simulink model "Robot"  (R2018a)
settings: Solver=VariableStepAuto  StartTime=0.0  StopTime=inf  FixedStep=1e-4  RelTol=1e-3  EnableMultiTasking=on
values from neighbouring files (symbols this model uses):
  CM730_acc_center = (4 * 9.80665)    (= 39.2266)    [CM730.m]
  CM730_acc_gain = 512 / CM730_acc_center    (= 13.0523675261)    [CM730.m]
  CM730_gyro_center = (1600 / 360 * 2 * pi)    (= 27.9252680319)    [CM730.m]
  CM730_gyro_gain = 512 / CM730_gyro_center    (= 18.3346494442)    [CM730.m]
  CM730_sample_time = 1e-3    (= 0.001)    [CM730.m]
  FSR_max = 254    [FSR.m]
  FSR_no_load = 255    [FSR.m]
  FSR_sample_time = 0.001    [FSR.m]
  FSR_scale = 1000    [FSR.m]
  g = 0    [Euler.m]
  MX106_Te = 1/1000    (= 0.001)    [MX106_init.m]
  MX28_inertia = 9e-8 * MX28_reduction^2    (= 0.0033385284)    [MX28_init.m]
  MX28_Te = 1/1000    (= 0.001)    [MX28_init.m]
  posZero_ID1 = posZero(1)    [Robot_init.m]
  posZero_ID10 = posZero(14)    [Robot_init.m]
  posZero_ID11 = posZero(9)    [Robot_init.m]
  posZero_ID12 = posZero(15)    [Robot_init.m]
  posZero_ID13 = posZero(10)    [Robot_init.m]
  posZero_ID14 = posZero(16)    [Robot_init.m]
  posZero_ID15 = posZero(11)    [Robot_init.m]
  posZero_ID16 = posZero(17)    [Robot_init.m]
  posZero_ID17 = posZero(12)    [Robot_init.m]
  posZero_ID18 = posZero(18)    [Robot_init.m]
  posZero_ID19 = posZero(19)    [Robot_init.m]
  posZero_ID2 = posZero(4)    [Robot_init.m]
  posZero_ID20 = posZero(20)    [Robot_init.m]
  posZero_ID3 = posZero(2)    [Robot_init.m]
  posZero_ID4 = posZero(5)    [Robot_init.m]
  posZero_ID5 = posZero(3)    [Robot_init.m]
  posZero_ID6 = posZero(6)    [Robot_init.m]
  posZero_ID7 = posZero(7)    [Robot_init.m]
  posZero_ID8 = posZero(13)    [Robot_init.m]
  posZero_ID9 = posZero(8)    [Robot_init.m]
  robot_chest_mass = 2385.0    (= 2385)    [Robot_init.m]
  robot_floor_friction_coeff = 0.6    [Robot_init.m]
  robot_floor_position_gain = -1e5    (= -100000)    [Robot_init.m]
  robot_floor_speed_gain = -1e3    (= -1000)    [Robot_init.m]
  robot_gravity = [0 0 0]    [Robot_init.m]
  robot_head_mass = 177.69    [Robot_init.m]
  robot_hip1_mass = 49.00    (= 49)    [Robot_init.m]
  robot_left_ankle_mass = 360.00    (= 360)    [Robot_init.m]
  robot_left_foot_mass = 267.00    (= 267)    [Robot_init.m]
  robot_left_forearm_mass = 248.00    (= 248)    [Robot_init.m]
  robot_left_hip2_mass = 358.00    (= 358)    [Robot_init.m]
  robot_left_lower_leg_mass = 129.00    (= 129)    [Robot_init.m]
  robot_left_shoulder_mass = 39.00    (= 39)    [Robot_init.m]
  robot_left_thigh_mass = 1263.00    (= 1263)    [Robot_init.m]
  robot_left_upper_arm_mass = 247.00    (= 247)    [Robot_init.m]
  robot_neck_mass = 90    [Robot_init.m]
  robot_right_ankle_mass = 360.00    (= 360)    [Robot_init.m]
  robot_right_foot_mass = 267.00    (= 267)    [Robot_init.m]
  robot_right_forearm_mass = 248.00    (= 248)    [Robot_init.m]
  robot_right_hip2_mass = 358.00    (= 358)    [Robot_init.m]
  robot_right_lower_leg_mass = 129.00    (= 129)    [Robot_init.m]
  robot_right_shoulder_mass = 39.00    (= 39)    [Robot_init.m]
  robot_right_thigh_mass = 263.00    (= 263)    [Robot_init.m]
  robot_right_upper_arm_mass = 247.00    (= 247)    [Robot_init.m]
  X = get(hObject,'Value')    [gui_kine.m]
  Y = get(hObject,'Value')    [gui_kine.m]
  Z = get(hObject,'Value')    [gui_kine.m]
libraries: sm_lib x167, fl_lib x128, nesl_utility x77, dspindex x1
(part 6 of 7)

== system Robot/Robot simulation/Right Leg/Right Knee (13) ==
  Inertia : sm_lib/Body Elements/Inertia  InertiaType=Custom  Mass=1  MassUnits=g  CenterOfMass=[0 0 0]  CenterOfMassUnits=m  MomentsOfInertia=[0 0 MX28_inertia]  MomentsOfInertiaUnits=kg*m^2  ProductsOfInertia=[0 0 0]  ProductsOfInertiaUnits=kg*m^2  GraphicType=Marker  MarkerShape=Inertia  MarkerSize=20  GraphicVisPropType=SimpleVisualProperties  GraphicDiffuseColor=[0.5 0.5 0.5]  GraphicSpecularColor=[0.5 0.5 0.5 1.0]  GraphicAmbientColor=[0.15 0.15 0.15 1.0]  GraphicEmissiveColor=[0.0 0.0 0.0 1.0]  GraphicShininess=75  GraphicOpacity=1.0
  MX106 Command : DataStoreRead  DataStoreName=MX106_ID13  SampleTime=MX106_Te  DataStoreElements=MX106_ID13.CW_angle_limit#MX106_ID13.CCW_angle_limit#MX106_ID13.torque_enable#MX106_ID13.D_gain#MX106_ID13.I_gain#MX106_ID13.P_gain#MX106_ID13.goal_position#MX106_ID13.moving_speed#MX106_ID13.torque_limit
  MX106 State : DataStoreWrite  DataStoreName=MX106_ID13  DataStoreElements=MX106_ID13.present_position#MX106_ID13.present_speed#MX106_ID13.present_load#MX106_ID13.moving#MX106_ID13.pwm
  Model : ModelReference  ModelNameDialog=MX106.slx  SimulationMode=Normal  ModelReferenceVersion=1.67
  Position converter : nesl_utility/PS-Simulink Converter  PhysicalDomain=network_engine_domain  SubClassName=ps_output  LeftPortType=input  RightPortType=output  PseudoPeriodic=off  Frequencies=[]  Unit=rad  AffineConversion=off
  Revolute Joint : sm_lib/Joints/Revolute Joint  SenseConstraintForce=off  SenseConstraintForceX=off  SenseConstraintForceY=off  SenseConstraintForceZ=off  SenseConstraintTorque=off  SenseConstraintTorqueX=off  SenseConstraintTorqueY=off  SenseConstraintTorqueZ=off  SenseTotalForce=off  SenseTotalForceX=off  SenseTotalForceY=off  SenseTotalForceZ=off  SenseTotalTorque=off  SenseTotalTorqueX=off  SenseTotalTorqueY=off  SenseTotalTorqueZ=off  CompositeWrenchDir=FollowerOnBase  CompositeWrenchFrame=BaseFrame  EquilibriumPosition=0  EquilibriumPositionUnits=deg  SpringStiffness=0  SpringStiffnessUnits=N*m/deg  DampingCoefficient=MX28_lub_friction  DampingCoefficientUnits=N*m/(rad/s)  TorqueActuationMode=InputTorque  MotionActuationMode=ComputedMotion  SensePosition=on  SenseVelocity=on  SenseAcceleration=off  SenseTorqueForce=off  PositionTargetSpecify=on  PositionTargetPriority=High  PositionTargetValue=MX28_init_position  PositionTargetValueUnits=rad  VelocityTargetSpecify=on  VelocityTargetPriority=High  VelocityTargetValue=MX28_init_speed  VelocityTargetValueUnits=rad/s
  Speed converter : nesl_utility/PS-Simulink Converter  PhysicalDomain=network_engine_domain  SubClassName=ps_output  LeftPortType=input  RightPortType=output  PseudoPeriodic=off  Frequencies=[]  Unit=rad/s  AffineConversion=off
  Torque converter : nesl_utility/Simulink-PS Converter  PhysicalDomain=network_engine_domain  SubClassName=ps_input  LeftPortType=input  RightPortType=output  PseudoPeriodic=off  Frequencies=[]  NoiseDistribution=none  NoiseParameters=[]  Unit=N*m  AffineConversion=off  FilteringAndDerivatives=zero  SimscapeFilterOrder=1  InputFilterTimeConstant=0.001  UdotUserProvided=1
  Base : PMIOPort  Side=Left
  Axis : PMIOPort  Port=2  Side=Right
  wires:
  Model/4 -> MX106 State/3
  Model/2 -> MX106 State/1
  Model/5 -> MX106 State/4
  Model/3 -> MX106 State/2
  MX106 Command/3 -> Model/5
  MX106 Command/6 -> Model/8
  MX106 Command/4 -> Model/6
  MX106 Command/5 -> Model/7
  MX106 Command/7 -> Model/9
  MX106 Command/2 -> Model/4
  MX106 Command/1 -> Model/3
  Position converter/1 -> Model/2
  Speed converter/1 -> Model/1
  Model/6 -> MX106 State/5
  MX106 Command/8 -> Model/10
  MX106 Command/9 -> Model/11
  Model/1 -> Torque converter/1
  connections:
  Axis/RConn1 -- Revolute Joint/RConn1 -- Inertia/RConn1
  Revolute Joint/LConn1 -- Base/RConn1
  Revolute Joint/RConn3 -- Speed converter/LConn1
  Revolute Joint/RConn2 -- Position converter/LConn1
  Revolute Joint/LConn2 -- Torque converter/RConn1

== system Robot/Robot simulation/Right Leg/Right Lower Leg ==
  Right Lower Leg Axis to Right Ankle Axis : sm_lib/Frames and Transforms/Rigid Transform  TranslationMethod=Cartesian  TranslationStandardOffset=0  TranslationLengthUnit=mm  TranslationStandardAxis=+Z  TranslationCartesianOffset=robot_right_lower_leg_to_right_ankle_tra  TranslationROffset=0  TranslationROffsetUnits=m  TranslationZOffset=0  TranslationZOffsetUnits=m  TranslationThetaOffset=0  TranslationThetaOffsetUnits=deg  RotationMethod=RotationMatrix  RotationAngleUnits=deg  RotationStandardAxis=+Z  RotationAngle=0  RotationArbitraryAxis=[0 0 1]  FollAlignAxisA=+X  BaseAlignAxisA=+Y  FollAlignAxisB=+Y  BaseAlignAxisB=+Z  RotationSequenceAxes=FollowerAxes  RotationSequence=XYX  RotationSequenceAngles=[0 0 0]  RotationSequenceAnglesUnits=deg  RotationMatrix=robot_right_lower_leg_to_right_ankle_rot
  Solid : sm_lib/Body Elements/Solid  InertiaType=Custom  Mass=robot_right_lower_leg_mass  MassUnits=g  CenterOfMass=robot_right_lower_leg_to_center_mass  CenterOfMassUnits=mm  MomentsOfInertia=robot_right_lower_leg_moment_inertia  MomentsOfInertiaUnits=g*mm^2  ProductsOfInertia=robot_right_lower_leg_product_inertia  ProductsOfInertiaUnits=g*mm^2  DensityBased=on  Density=1000  DensityUnits=kg/(m^3)  DoExposeReferenceFrame=on  SerializedFrames=<Frames/>  GraphicType=FromGeometry  MarkerShape=Sphere  MarkerSize=10  MarkerSizeUnits=m  GraphicVisPropType=SimpleVisualProperties  GraphicDiffuseColor=[0.5 0.5 0.5]  GraphicSpecularColor=[0.5 0.5 0.5 1.0]  GraphicAmbientColor=[0.15 0.15 0.15 1.0]  GraphicEmissiveColor=[0.0 0.0 0.0 1.0]  GraphicShininess=75  GraphicOpacity=1.0  GeometryShape=FromFile  RectangleSize=[1 1]  RectangleSizeUnits=m  BrickDimensions=[1 1 1]  BrickDimensionUnits=m  CylinderRadius=1  CylinderRadiusUnits=m  CylinderLength=1  CylinderLengthUnits=m  SphereRadius=1  SphereRadiusUnits=m  EllipsoidRadii=[1 1 1]  EllipsoidRadiiUnits=m  ExtrusionCrossSection=[1 1; -1 1; -1 -1; 1 -1]  ExtrusionCrossSectionUnits=m  ExtrusionLength=1  ExtrusionLengthUnits=m  PolygonNumSides=3  PolygonOuterRadius=1  PolygonOuterRadiusUnits=m  ExtGeomFileType=STL  ExtGeomFileName=\STL\Right_Lower_Leg.STL  ExtGeomFileUnits=mm  RevolutionCrossSection=[1 1; 1 -1; 2 -1; 2 1]  RevolutionCrossSectionUnits=m  RevolutionExtent=Full  RevolutionAngle=180  RevolutionAngleUnits=deg
  Right Knee : PMIOPort  Side=Left
  Right Ankle Pitch : PMIOPort  Port=2  Side=Right
  connections:
  Solid/RConn1 -- Right Lower Leg Axis to Right Ankle Axis/LConn1 -- Right Knee/RConn1
  Right Ankle Pitch/RConn1 -- Right Lower Leg Axis to Right Ankle Axis/RConn1

== system Robot/Robot simulation/Right Leg/Right Thigh ==
  Right Hip Pitch Axis to Right Lower Leg Base : sm_lib/Frames and Transforms/Rigid Transform  TranslationMethod=Cartesian  TranslationStandardOffset=0  TranslationLengthUnit=mm  TranslationStandardAxis=+Z  TranslationCartesianOffset=robot_right_thigh_to_right_lower_leg_tra  TranslationROffset=0  TranslationROffsetUnits=m  TranslationZOffset=0  TranslationZOffsetUnits=m  TranslationThetaOffset=0  TranslationThetaOffsetUnits=deg  RotationMethod=RotationMatrix  RotationAngleUnits=deg  RotationStandardAxis=+Z  RotationAngle=0  RotationArbitraryAxis=[0 0 1]  FollAlignAxisA=+X  BaseAlignAxisA=+Y  FollAlignAxisB=+Y  BaseAlignAxisB=+Z  RotationSequenceAxes=FollowerAxes  RotationSequence=XYX  RotationSequenceAngles=[0 0 0]  RotationSequenceAnglesUnits=deg  RotationMatrix=robot_right_thigh_to_right_lower_leg_rot
  Solid : sm_lib/Body Elements/Solid  InertiaType=Custom  Mass=robot_right_thigh_mass  MassUnits=g  CenterOfMass=robot_right_thigh_to_center_mass  CenterOfMassUnits=mm  MomentsOfInertia=robot_right_thigh_moment_inertia  MomentsOfInertiaUnits=g*mm^2  ProductsOfInertia=robot_right_thigh_product_inertia  ProductsOfInertiaUnits=g*mm^2  DensityBased=on  Density=1000  DensityUnits=kg/(m^3)  DoExposeReferenceFrame=on  SerializedFrames=<Frames/>  GraphicType=FromGeometry  MarkerShape=Sphere  MarkerSize=10  MarkerSizeUnits=m  GraphicVisPropType=SimpleVisualProperties  GraphicDiffuseColor=[0.5 0.5 0.5]  GraphicSpecularColor=[0.5 0.5 0.5 1.0]  GraphicAmbientColor=[0.15 0.15 0.15 1.0]  GraphicEmissiveColor=[0.0 0.0 0.0 1.0]  GraphicShininess=75  GraphicOpacity=1.0  GeometryShape=FromFile  RectangleSize=[1 1]  RectangleSizeUnits=m  BrickDimensions=[1 1 1]  BrickDimensionUnits=m  CylinderRadius=1  CylinderRadiusUnits=m  CylinderLength=1  CylinderLengthUnits=m  SphereRadius=1  SphereRadiusUnits=m  EllipsoidRadii=[1 1 1]  EllipsoidRadiiUnits=m  ExtrusionCrossSection=[1 1; -1 1; -1 -1; 1 -1]  ExtrusionCrossSectionUnits=m  ExtrusionLength=1  ExtrusionLengthUnits=m  PolygonNumSides=3  PolygonOuterRadius=1  PolygonOuterRadiusUnits=m  ExtGeomFileType=STL  ExtGeomFileName=\STL\Right_Thigh.STL  ExtGeomFileUnits=mm  RevolutionCrossSection=[1 1; 1 -1; 2 -1; 2 1]  RevolutionCrossSectionUnits=m  RevolutionExtent=Full  RevolutionAngle=180  RevolutionAngleUnits=deg
  Right Hip Pitch : PMIOPort  Side=Left
  Right Knee : PMIOPort  Port=2  Side=Right
  connections:
  Right Hip Pitch Axis to Right Lower Leg Base/LConn1 -- Right Hip Pitch/RConn1 -- Solid/RConn1
  Right Knee/RConn1 -- Right Hip Pitch Axis to Right Lower Leg Base/RConn1

== system Robot/Robot simulation/Left Leg/Floor model/Floor Model Back Left ==
  6-DOF Joint1 : sm_lib/Joints/6-DOF Joint  SenseConstraintForce=off  SenseConstraintForceX=off  SenseConstraintForceY=off  SenseConstraintForceZ=off  SenseConstraintTorque=off  SenseConstraintTorqueX=off  SenseConstraintTorqueY=off  SenseConstraintTorqueZ=off  SenseTotalForce=off  SenseTotalForceX=off  SenseTotalForceY=off  SenseTotalForceZ=off  SenseTotalTorque=off  SenseTotalTorqueX=off  SenseTotalTorqueY=off  SenseTotalTorqueZ=off  CompositeWrenchDir=FollowerOnBase  CompositeWrenchFrame=BaseFrame  PxEquilibriumPosition=0  PxEquilibriumPositionUnits=m  PxSpringStiffness=0  PxSpringStiffnessUnits=N/m  PxDampingCoefficient=0  PxDampingCoefficientUnits=N/(m/s)  PxTorqueActuationMode=InputTorque  PxMotionActuationMode=ComputedMotion  PxSensePosition=off  PxSenseVelocity=on  PxSenseAcceleration=off  PxSenseTorqueForce=off  PxPositionTargetSpecify=off  PxPositionTargetPriority=High  PxPositionTargetValue=0  PxPositionTargetValueUnits=m  PxVelocityTargetSpecify=off  PxVelocityTargetPriority=High  PxVelocityTargetValue=0  PxVelocityTargetValueUnits=m/s  PyEquilibriumPosition=0  PyEquilibriumPositionUnits=m  PySpringStiffness=0  PySpringStiffnessUnits=N/m  PyDampingCoefficient=0  PyDampingCoefficientUnits=N/(m/s)  PyTorqueActuationMode=InputTorque  PyMotionActuationMode=ComputedMotion  PySensePosition=off  PySenseVelocity=on  PySenseAcceleration=off  PySenseTorqueForce=off  PyPositionTargetSpecify=off  PyPositionTargetPriority=High  PyPositionTargetValue=0  PyPositionTargetValueUnits=m  PyVelocityTargetSpecify=off  PyVelocityTargetPriority=High  PyVelocityTargetValue=0  PyVelocityTargetValueUnits=m/s  PzEquilibriumPosition=0  PzEquilibriumPositionUnits=m  PzSpringStiffness=0  PzSpringStiffnessUnits=N/m  PzDampingCoefficient=0  PzDampingCoefficientUnits=N/(m/s)  PzTorqueActuationMode=InputTorque  PzMotionActuationMode=ComputedMotion  PzSensePosition=on  PzSenseVelocity=on  PzSenseAcceleration=off  PzSenseTorqueForce=off  PzPositionTargetSpecify=off  PzPositionTargetPriority=High  PzPositionTargetValue=0  PzPositionTargetValueUnits=m  PzVelocityTargetSpecify=off  PzVelocityTargetPriority=High  PzVelocityTargetValue=0  PzVelocityTargetValueUnits=m/s  SphDefPosRotationMethod=None  SphDefPosRotationAngleUnits=deg  SphDefPosRotationStandardAxis=+Z  SphDefPosRotationAngle=0.0  SphDefPosRotationArbitraryAxis=[0 0 1]  SphDefPosFollAlignAxisA=+X  SphDefPosBaseAlignAxisA=+Y  SphDefPosFollAlignAxisB=+Y  SphDefPosBaseAlignAxisB=+Z  SphDefPosRotationSequenceAxes=FollowerAxes  SphDefPosRotationSequence=XYX  SphDefPosRotationSequenceAngles=[0 0 0]  SphDefPosRotationSequenceAnglesUnits=deg  SphDefPosRotationMatrix=[1 0 0; 0 1 0; 0 0 1]  SphEqPosRotationMethod=None  SphEqPosRotationAngleUnits=deg  SphEqPosRotationStandardAxis=+Z  SphEqPosRotationAngle=0.0  SphEqPosRotationArbitraryAxis=[0 0 1]  SphEqPosFollAlignAxisA=+X  SphEqPosBaseAlignAxisA=+Y  SphEqPosFollAlignAxisB=+Y  SphEqPosBaseAlignAxisB=+Z  SphEqPosRotationSequenceAxes=FollowerAxes  SphEqPosRotationSequence=XYX  SphEqPosRotationSequenceAngles=[0 0 0]  SphEqPosRotationSequenceAnglesUnits=deg  SphEqPosRotationMatrix=[1 0 0; 0 1 0; 0 0 1]  SphSpringStiffness=0  SphSpringStiffnessUnits=N*m/deg  SphDampingCoefficient=0  SphDampingCoefficientUnits=N*m/(deg/s)  SphActuateTorqueX=off  SphActuateTorqueY=off  SphActuateTorqueZ=off  SphActuateTorque=off  SphTorqueActuationMode=NoTorque  SphMotionActuationMode=ComputedMotion  SphActuationFrame=BaseFrame  SphSensePosition=off  SphSenseVelocityX=off  SphSenseVelocityY=off  SphSenseVelocityZ=off  SphSenseVelocity=off  SphSenseAccelerationX=off  SphSenseAccelerationY=off  SphSenseAccelerationZ=off  SphSenseAcceleration=off  SphSenseTorqueX=off  SphSenseTorqueY=off  SphSenseTorqueZ=off  SphSenseTorqueForce=off  SphSensingFrame=BaseFrame  SphPositionTargetRotationMethod=None  SphPositionTargetRotationAngleUnits=deg  SphPositionTargetRotationStandardAxis=+Z  SphPositionTargetRotationAngle=0.0  SphPositionTargetRotationArbitraryAxis=[0 0 1]  SphPositionTargetFollAlignAxisA=+X  SphPositionTargetBaseAlignAxisA=+Y  SphPositionTargetFollAlignAxisB=+Y  SphPositionTargetBaseAlignAxisB=+Z  SphPositionTargetRotationSequenceAxes=FollowerAxes  SphPositionTargetRotationSequence=XYX  SphPositionTargetRotationSequenceAngles=[0 0 0]  SphPositionTargetRotationSequenceAnglesUnits=deg  SphPositionTargetRotationMatrix=[1 0 0; 0 1 0; 0 0 1]  SphPositionTargetSpecify=off  SphPositionTargetPriority=High  SphVelocityTargetValue=[0 0 0]  SphVelocityTargetValueUnits=deg/s  SphVelocityTargetSpecify=off  SphVelocityTargetPriority=High  SphVelocityTargetInFollowerFrame=on
  Friction coeff : fl_lib/Physical Signals/Functions/PS Gain  gain=robot_floor_friction_coeff
  No friction : fl_lib/Physical Signals/Sources/PS Constant  constant=0
  PS Abs : fl_lib/Physical Signals/Nonlinear Operators/PS Abs
      settings: SourceProductName=Simscape  SourceProductBaseCode=SS
  PS-Simulink Converter : nesl_utility/PS-Simulink Converter  PhysicalDomain=network_engine_domain  SubClassName=ps_output  LeftPortType=input  RightPortType=output  PseudoPeriodic=off  Frequencies=[]  Unit=N  AffineConversion=off
  Saturation : Saturate  UpperLimit=+inf  LowerLimit=0
  Unary minus : fl_lib/Physical Signals/Functions/PS Gain  gain=-1
  X Lower Bound : fl_lib/Physical Signals/Nonlinear Operators/PS Max
      settings: SourceProductName=Simscape  SourceProductBaseCode=SS
  X Speed Gain : fl_lib/Physical Signals/Functions/PS Gain  gain=robot_floor_speed_gain
  X Switch : fl_lib/Physical Signals/Nonlinear Operators/PS Switch  Threshold=0
      settings: SourceProductName=Simscape  SourceProductBaseCode=SS
  X Upper Bound : fl_lib/Physical Signals/Nonlinear Operators/PS Min
      settings: SourceProductName=Simscape  SourceProductBaseCode=SS
  Y Lower Bound : fl_lib/Physical Signals/Nonlinear Operators/PS Max
      settings: SourceProductName=Simscape  SourceProductBaseCode=SS
  Y Speed Gain : fl_lib/Physical Signals/Functions/PS Gain  gain=robot_floor_speed_gain
  Y Switch : fl_lib/Physical Signals/Nonlinear Operators/PS Switch  Threshold=0
      settings: SourceProductName=Simscape  SourceProductBaseCode=SS
  Y Upper Bound : fl_lib/Physical Signals/Nonlinear Operators/PS Min
      settings: SourceProductName=Simscape  SourceProductBaseCode=SS
  Z Add : fl_lib/Physical Signals/Functions/PS Add
  Z Position Gain : fl_lib/Physical Signals/Functions/PS Gain  gain=robot_floor_position_gain
  Z Speed Gain : fl_lib/Physical Signals/Functions/PS Gain  gain=robot_floor_speed_gain
  Z Switch : fl_lib/Physical Signals/Nonlinear Operators/PS Switch  Threshold=0
      settings: SourceProductName=Simscape  SourceProductBaseCode=SS
  Contact : PMIOPort  Side=Left
  Floor : PMIOPort  Port=2  Side=Right
  Z force : Outport
  wires:
  PS-Simulink Converter/1 -> Saturation/1
  Saturation/1 -> Z force/1
  connections:
  Floor/RConn1 -- 6-DOF Joint1/LConn1
  6-DOF Joint1/RConn1 -- Contact/RConn1
  No friction/RConn1 -- Y Switch/LConn1 -- Z Switch/LConn1 -- X Switch/LConn1
  Z Position Gain/RConn1 -- Z Add/LConn1
  Z Switch/LConn3 -- Z Add/RConn1 -- Friction coeff/LConn1 -- PS-Simulink Converter/LConn1
  Z Speed Gain/RConn1 -- Z Add/LConn2
  6-DOF Joint1/RConn5 -- Z Speed Gain/LConn1
  6-DOF Joint1/LConn4 -- Z Switch/RConn1
  Z Switch/LConn2 -- Z Position Gain/LConn1 -- 6-DOF Joint1/RConn4 -- X Switch/LConn2 -- Y Switch/LConn2
  Y Switch/RConn1 -- 6-DOF Joint1/LConn3
  Y Speed Gain/LConn1 -- 6-DOF Joint1/RConn3
  PS Abs/LConn1 -- Friction coeff/RConn1
  PS Abs/RConn1 -- Unary minus/LConn1 -- X Upper Bound/LConn2 -- Y Upper Bound/LConn2
  Y Upper Bound/RConn1 -- Y Lower Bound/LConn1
  Y Lower Bound/LConn2 -- Unary minus/RConn1 -- X Lower Bound/LConn2
  Y Lower Bound/RConn1 -- Y Switch/LConn3
  Y Upper Bound/LConn1 -- Y Speed Gain/RConn1
  X Speed Gain/LConn1 -- 6-DOF Joint1/RConn2
  X Upper Bound/LConn1 -- X Speed Gain/RConn1
  X Lower Bound/LConn1 -- X Upper Bound/RConn1
  X Switch/LConn3 -- X Lower Bound/RConn1
  X Switch/RConn1 -- 6-DOF Joint1/LConn2

== system Robot/Robot simulation/Left Leg/Floor model/Floor Model Back Right ==
  6-DOF Joint1 : sm_lib/Joints/6-DOF Joint  SenseConstraintForce=off  SenseConstraintForceX=off  SenseConstraintForceY=off  SenseConstraintForceZ=off  SenseConstraintTorque=off  SenseConstraintTorqueX=off  SenseConstraintTorqueY=off  SenseConstraintTorqueZ=off  SenseTotalForce=off  SenseTotalForceX=off  SenseTotalForceY=off  SenseTotalForceZ=off  SenseTotalTorque=off  SenseTotalTorqueX=off  SenseTotalTorqueY=off  SenseTotalTorqueZ=off  CompositeWrenchDir=FollowerOnBase  CompositeWrenchFrame=BaseFrame  PxEquilibriumPosition=0  PxEquilibriumPositionUnits=m  PxSpringStiffness=0  PxSpringStiffnessUnits=N/m  PxDampingCoefficient=0  PxDampingCoefficientUnits=N/(m/s)  PxTorqueActuationMode=InputTorque  PxMotionActuationMode=ComputedMotion  PxSensePosition=off  PxSenseVelocity=on  PxSenseAcceleration=off  PxSenseTorqueForce=off  PxPositionTargetSpecify=off  PxPositionTargetPriority=High  PxPositionTargetValue=0  PxPositionTargetValueUnits=m  PxVelocityTargetSpecify=off  PxVelocityTargetPriority=High  PxVelocityTargetValue=0  PxVelocityTargetValueUnits=m/s  PyEquilibriumPosition=0  PyEquilibriumPositionUnits=m  PySpringStiffness=0  PySpringStiffnessUnits=N/m  PyDampingCoefficient=0  PyDampingCoefficientUnits=N/(m/s)  PyTorqueActuationMode=InputTorque  PyMotionActuationMode=ComputedMotion  PySensePosition=off  PySenseVelocity=on  PySenseAcceleration=off  PySenseTorqueForce=off  PyPositionTargetSpecify=off  PyPositionTargetPriority=High  PyPositionTargetValue=0  PyPositionTargetValueUnits=m  PyVelocityTargetSpecify=off  PyVelocityTargetPriority=High  PyVelocityTargetValue=0  PyVelocityTargetValueUnits=m/s  PzEquilibriumPosition=0  PzEquilibriumPositionUnits=m  PzSpringStiffness=0  PzSpringStiffnessUnits=N/m  PzDampingCoefficient=0  PzDampingCoefficientUnits=N/(m/s)  PzTorqueActuationMode=InputTorque  PzMotionActuationMode=ComputedMotion  PzSensePosition=on  PzSenseVelocity=on  PzSenseAcceleration=off  PzSenseTorqueForce=off  PzPositionTargetSpecify=off  PzPositionTargetPriority=High  PzPositionTargetValue=0  PzPositionTargetValueUnits=m  PzVelocityTargetSpecify=off  PzVelocityTargetPriority=High  PzVelocityTargetValue=0  PzVelocityTargetValueUnits=m/s  SphDefPosRotationMethod=None  SphDefPosRotationAngleUnits=deg  SphDefPosRotationStandardAxis=+Z  SphDefPosRotationAngle=0.0  SphDefPosRotationArbitraryAxis=[0 0 1]  SphDefPosFollAlignAxisA=+X  SphDefPosBaseAlignAxisA=+Y  SphDefPosFollAlignAxisB=+Y  SphDefPosBaseAlignAxisB=+Z  SphDefPosRotationSequenceAxes=FollowerAxes  SphDefPosRotationSequence=XYX  SphDefPosRotationSequenceAngles=[0 0 0]  SphDefPosRotationSequenceAnglesUnits=deg  SphDefPosRotationMatrix=[1 0 0; 0 1 0; 0 0 1]  SphEqPosRotationMethod=None  SphEqPosRotationAngleUnits=deg  SphEqPosRotationStandardAxis=+Z  SphEqPosRotationAngle=0.0  SphEqPosRotationArbitraryAxis=[0 0 1]  SphEqPosFollAlignAxisA=+X  SphEqPosBaseAlignAxisA=+Y  SphEqPosFollAlignAxisB=+Y  SphEqPosBaseAlignAxisB=+Z  SphEqPosRotationSequenceAxes=FollowerAxes  SphEqPosRotationSequence=XYX  SphEqPosRotationSequenceAngles=[0 0 0]  SphEqPosRotationSequenceAnglesUnits=deg  SphEqPosRotationMatrix=[1 0 0; 0 1 0; 0 0 1]  SphSpringStiffness=0  SphSpringStiffnessUnits=N*m/deg  SphDampingCoefficient=0  SphDampingCoefficientUnits=N*m/(deg/s)  SphActuateTorqueX=off  SphActuateTorqueY=off  SphActuateTorqueZ=off  SphActuateTorque=off  SphTorqueActuationMode=NoTorque  SphMotionActuationMode=ComputedMotion  SphActuationFrame=BaseFrame  SphSensePosition=off  SphSenseVelocityX=off  SphSenseVelocityY=off  SphSenseVelocityZ=off  SphSenseVelocity=off  SphSenseAccelerationX=off  SphSenseAccelerationY=off  SphSenseAccelerationZ=off  SphSenseAcceleration=off  SphSenseTorqueX=off  SphSenseTorqueY=off  SphSenseTorqueZ=off  SphSenseTorqueForce=off  SphSensingFrame=BaseFrame  SphPositionTargetRotationMethod=None  SphPositionTargetRotationAngleUnits=deg  SphPositionTargetRotationStandardAxis=+Z  SphPositionTargetRotationAngle=0.0  SphPositionTargetRotationArbitraryAxis=[0 0 1]  SphPositionTargetFollAlignAxisA=+X  SphPositionTargetBaseAlignAxisA=+Y  SphPositionTargetFollAlignAxisB=+Y  SphPositionTargetBaseAlignAxisB=+Z  SphPositionTargetRotationSequenceAxes=FollowerAxes  SphPositionTargetRotationSequence=XYX  SphPositionTargetRotationSequenceAngles=[0 0 0]  SphPositionTargetRotationSequenceAnglesUnits=deg  SphPositionTargetRotationMatrix=[1 0 0; 0 1 0; 0 0 1]  SphPositionTargetSpecify=off  SphPositionTargetPriority=High  SphVelocityTargetValue=[0 0 0]  SphVelocityTargetValueUnits=deg/s  SphVelocityTargetSpecify=off  SphVelocityTargetPriority=High  SphVelocityTargetInFollowerFrame=on
  Friction coeff : fl_lib/Physical Signals/Functions/PS Gain  gain=robot_floor_friction_coeff
  No friction : fl_lib/Physical Signals/Sources/PS Constant  constant=0
  PS Abs : fl_lib/Physical Signals/Nonlinear Operators/PS Abs
      settings: SourceProductName=Simscape  SourceProductBaseCode=SS
  PS-Simulink Converter : nesl_utility/PS-Simulink Converter  PhysicalDomain=network_engine_domain  SubClassName=ps_output  LeftPortType=input  RightPortType=output  PseudoPeriodic=off  Frequencies=[]  Unit=N  AffineConversion=off
  Saturation : Saturate  UpperLimit=+inf  LowerLimit=0
  Unary minus : fl_lib/Physical Signals/Functions/PS Gain  gain=-1
  X Lower Bound : fl_lib/Physical Signals/Nonlinear Operators/PS Max
      settings: SourceProductName=Simscape  SourceProductBaseCode=SS
  X Speed Gain : fl_lib/Physical Signals/Functions/PS Gain  gain=robot_floor_speed_gain
  X Switch : fl_lib/Physical Signals/Nonlinear Operators/PS Switch  Threshold=0
      settings: SourceProductName=Simscape  SourceProductBaseCode=SS
  X Upper Bound : fl_lib/Physical Signals/Nonlinear Operators/PS Min
      settings: SourceProductName=Simscape  SourceProductBaseCode=SS
  Y Lower Bound : fl_lib/Physical Signals/Nonlinear Operators/PS Max
      settings: SourceProductName=Simscape  SourceProductBaseCode=SS
  Y Speed Gain : fl_lib/Physical Signals/Functions/PS Gain  gain=robot_floor_speed_gain
  Y Switch : fl_lib/Physical Signals/Nonlinear Operators/PS Switch  Threshold=0
      settings: SourceProductName=Simscape  SourceProductBaseCode=SS
  Y Upper Bound : fl_lib/Physical Signals/Nonlinear Operators/PS Min
      settings: SourceProductName=Simscape  SourceProductBaseCode=SS
  Z Add : fl_lib/Physical Signals/Functions/PS Add
  Z Position Gain : fl_lib/Physical Signals/Functions/PS Gain  gain=robot_floor_position_gain
  Z Speed Gain : fl_lib/Physical Signals/Functions/PS Gain  gain=robot_floor_speed_gain
  Z Switch : fl_lib/Physical Signals/Nonlinear Operators/PS Switch  Threshold=0
      settings: SourceProductName=Simscape  SourceProductBaseCode=SS
  Contact : PMIOPort  Side=Left
  Floor : PMIOPort  Port=2  Side=Right
  Z force : Outport
  wires:
  PS-Simulink Converter/1 -> Saturation/1
  Saturation/1 -> Z force/1
  connections:
  Floor/RConn1 -- 6-DOF Joint1/LConn1
  6-DOF Joint1/RConn1 -- Contact/RConn1
  No friction/RConn1 -- Y Switch/LConn1 -- Z Switch/LConn1 -- X Switch/LConn1
  Z Position Gain/RConn1 -- Z Add/LConn1
  Z Switch/LConn3 -- Z Add/RConn1 -- Friction coeff/LConn1 -- PS-Simulink Converter/LConn1
  Z Speed Gain/RConn1 -- Z Add/LConn2
  6-DOF Joint1/RConn5 -- Z Speed Gain/LConn1
  6-DOF Joint1/LConn4 -- Z Switch/RConn1
  Z Switch/LConn2 -- Z Position Gain/LConn1 -- 6-DOF Joint1/RConn4 -- X Switch/LConn2 -- Y Switch/LConn2
  Y Switch/RConn1 -- 6-DOF Joint1/LConn3
  Y Speed Gain/LConn1 -- 6-DOF Joint1/RConn3
  PS Abs/LConn1 -- Friction coeff/RConn1
  PS Abs/RConn1 -- Unary minus/LConn1 -- X Upper Bound/LConn2 -- Y Upper Bound/LConn2
  Y Upper Bound/RConn1 -- Y Lower Bound/LConn1
  Y Lower Bound/LConn2 -- Unary minus/RConn1 -- X Lower Bound/LConn2
  Y Lower Bound/RConn1 -- Y Switch/LConn3
  Y Upper Bound/LConn1 -- Y Speed Gain/RConn1
  X Speed Gain/LConn1 -- 6-DOF Joint1/RConn2
  X Upper Bound/LConn1 -- X Speed Gain/RConn1
  X Lower Bound/LConn1 -- X Upper Bound/RConn1
  X Switch/LConn3 -- X Lower Bound/RConn1
  X Switch/RConn1 -- 6-DOF Joint1/LConn2

== system Robot/Robot simulation/Left Leg/Floor model/Floor Model Front Left ==
  6-DOF Joint1 : sm_lib/Joints/6-DOF Joint  SenseConstraintForce=off  SenseConstraintForceX=off  SenseConstraintForceY=off  SenseConstraintForceZ=off  SenseConstraintTorque=off  SenseConstraintTorqueX=off  SenseConstraintTorqueY=off  SenseConstraintTorqueZ=off  SenseTotalForce=off  SenseTotalForceX=off  SenseTotalForceY=off  SenseTotalForceZ=off  SenseTotalTorque=off  SenseTotalTorqueX=off  SenseTotalTorqueY=off  SenseTotalTorqueZ=off  CompositeWrenchDir=FollowerOnBase  CompositeWrenchFrame=BaseFrame  PxEquilibriumPosition=0  PxEquilibriumPositionUnits=m  PxSpringStiffness=0  PxSpringStiffnessUnits=N/m  PxDampingCoefficient=0  PxDampingCoefficientUnits=N/(m/s)  PxTorqueActuationMode=InputTorque  PxMotionActuationMode=ComputedMotion  PxSensePosition=off  PxSenseVelocity=on  PxSenseAcceleration=off  PxSenseTorqueForce=off  PxPositionTargetSpecify=off  PxPositionTargetPriority=High  PxPositionTargetValue=0  PxPositionTargetValueUnits=m  PxVelocityTargetSpecify=off  PxVelocityTargetPriority=High  PxVelocityTargetValue=0  PxVelocityTargetValueUnits=m/s  PyEquilibriumPosition=0  PyEquilibriumPositionUnits=m  PySpringStiffness=0  PySpringStiffnessUnits=N/m  PyDampingCoefficient=0  PyDampingCoefficientUnits=N/(m/s)  PyTorqueActuationMode=InputTorque  PyMotionActuationMode=ComputedMotion  PySensePosition=off  PySenseVelocity=on  PySenseAcceleration=off  PySenseTorqueForce=off  PyPositionTargetSpecify=off  PyPositionTargetPriority=High  PyPositionTargetValue=0  PyPositionTargetValueUnits=m  PyVelocityTargetSpecify=off  PyVelocityTargetPriority=High  PyVelocityTargetValue=0  PyVelocityTargetValueUnits=m/s  PzEquilibriumPosition=0  PzEquilibriumPositionUnits=m  PzSpringStiffness=0  PzSpringStiffnessUnits=N/m  PzDampingCoefficient=0  PzDampingCoefficientUnits=N/(m/s)  PzTorqueActuationMode=InputTorque  PzMotionActuationMode=ComputedMotion  PzSensePosition=on  PzSenseVelocity=on  PzSenseAcceleration=off  PzSenseTorqueForce=off  PzPositionTargetSpecify=off  PzPositionTargetPriority=High  PzPositionTargetValue=0  PzPositionTargetValueUnits=m  PzVelocityTargetSpecify=off  PzVelocityTargetPriority=High  PzVelocityTargetValue=0  PzVelocityTargetValueUnits=m/s  SphDefPosRotationMethod=None  SphDefPosRotationAngleUnits=deg  SphDefPosRotationStandardAxis=+Z  SphDefPosRotationAngle=0.0  SphDefPosRotationArbitraryAxis=[0 0 1]  SphDefPosFollAlignAxisA=+X  SphDefPosBaseAlignAxisA=+Y  SphDefPosFollAlignAxisB=+Y  SphDefPosBaseAlignAxisB=+Z  SphDefPosRotationSequenceAxes=FollowerAxes  SphDefPosRotationSequence=XYX  SphDefPosRotationSequenceAngles=[0 0 0]  SphDefPosRotationSequenceAnglesUnits=deg  SphDefPosRotationMatrix=[1 0 0; 0 1 0; 0 0 1]  SphEqPosRotationMethod=None  SphEqPosRotationAngleUnits=deg  SphEqPosRotationStandardAxis=+Z  SphEqPosRotationAngle=0.0  SphEqPosRotationArbitraryAxis=[0 0 1]  SphEqPosFollAlignAxisA=+X  SphEqPosBaseAlignAxisA=+Y  SphEqPosFollAlignAxisB=+Y  SphEqPosBaseAlignAxisB=+Z  SphEqPosRotationSequenceAxes=FollowerAxes  SphEqPosRotationSequence=XYX  SphEqPosRotationSequenceAngles=[0 0 0]  SphEqPosRotationSequenceAnglesUnits=deg  SphEqPosRotationMatrix=[1 0 0; 0 1 0; 0 0 1]  SphSpringStiffness=0  SphSpringStiffnessUnits=N*m/deg  SphDampingCoefficient=0  SphDampingCoefficientUnits=N*m/(deg/s)  SphActuateTorqueX=off  SphActuateTorqueY=off  SphActuateTorqueZ=off  SphActuateTorque=off  SphTorqueActuationMode=NoTorque  SphMotionActuationMode=ComputedMotion  SphActuationFrame=BaseFrame  SphSensePosition=off  SphSenseVelocityX=off  SphSenseVelocityY=off  SphSenseVelocityZ=off  SphSenseVelocity=off  SphSenseAccelerationX=off  SphSenseAccelerationY=off  SphSenseAccelerationZ=off  SphSenseAcceleration=off  SphSenseTorqueX=off  SphSenseTorqueY=off  SphSenseTorqueZ=off  SphSenseTorqueForce=off  SphSensingFrame=BaseFrame  SphPositionTargetRotationMethod=None  SphPositionTargetRotationAngleUnits=deg  SphPositionTargetRotationStandardAxis=+Z  SphPositionTargetRotationAngle=0.0  SphPositionTargetRotationArbitraryAxis=[0 0 1]  SphPositionTargetFollAlignAxisA=+X  SphPositionTargetBaseAlignAxisA=+Y  SphPositionTargetFollAlignAxisB=+Y  SphPositionTargetBaseAlignAxisB=+Z  SphPositionTargetRotationSequenceAxes=FollowerAxes  SphPositionTargetRotationSequence=XYX  SphPositionTargetRotationSequenceAngles=[0 0 0]  SphPositionTargetRotationSequenceAnglesUnits=deg  SphPositionTargetRotationMatrix=[1 0 0; 0 1 0; 0 0 1]  SphPositionTargetSpecify=off  SphPositionTargetPriority=High  SphVelocityTargetValue=[0 0 0]  SphVelocityTargetValueUnits=deg/s  SphVelocityTargetSpecify=off  SphVelocityTargetPriority=High  SphVelocityTargetInFollowerFrame=on
  Friction coeff : fl_lib/Physical Signals/Functions/PS Gain  gain=robot_floor_friction_coeff
  No friction : fl_lib/Physical Signals/Sources/PS Constant  constant=0
  PS Abs : fl_lib/Physical Signals/Nonlinear Operators/PS Abs
      settings: SourceProductName=Simscape  SourceProductBaseCode=SS
  PS-Simulink Converter : nesl_utility/PS-Simulink Converter  PhysicalDomain=network_engine_domain  SubClassName=ps_output  LeftPortType=input  RightPortType=output  PseudoPeriodic=off  Frequencies=[]  Unit=N  AffineConversion=off
  Saturation : Saturate  UpperLimit=+inf  LowerLimit=0
  Unary minus : fl_lib/Physical Signals/Functions/PS Gain  gain=-1
  X Lower Bound : fl_lib/Physical Signals/Nonlinear Operators/PS Max
      settings: SourceProductName=Simscape  SourceProductBaseCode=SS
  X Speed Gain : fl_lib/Physical Signals/Functions/PS Gain  gain=robot_floor_speed_gain
  X Switch : fl_lib/Physical Signals/Nonlinear Operators/PS Switch  Threshold=0
      settings: SourceProductName=Simscape  SourceProductBaseCode=SS
  X Upper Bound : fl_lib/Physical Signals/Nonlinear Operators/PS Min
      settings: SourceProductName=Simscape  SourceProductBaseCode=SS
  Y Lower Bound : fl_lib/Physical Signals/Nonlinear Operators/PS Max
      settings: SourceProductName=Simscape  SourceProductBaseCode=SS
  Y Speed Gain : fl_lib/Physical Signals/Functions/PS Gain  gain=robot_floor_speed_gain
  Y Switch : fl_lib/Physical Signals/Nonlinear Operators/PS Switch  Threshold=0
      settings: SourceProductName=Simscape  SourceProductBaseCode=SS
  Y Upper Bound : fl_lib/Physical Signals/Nonlinear Operators/PS Min
      settings: SourceProductName=Simscape  SourceProductBaseCode=SS
  Z Add : fl_lib/Physical Signals/Functions/PS Add
  Z Position Gain : fl_lib/Physical Signals/Functions/PS Gain  gain=robot_floor_position_gain
  Z Speed Gain : fl_lib/Physical Signals/Functions/PS Gain  gain=robot_floor_speed_gain
  Z Switch : fl_lib/Physical Signals/Nonlinear Operators/PS Switch  Threshold=0
      settings: SourceProductName=Simscape  SourceProductBaseCode=SS
  Contact : PMIOPort  Side=Left
  Floor : PMIOPort  Port=2  Side=Right
  Z force : Outport
  wires:
  PS-Simulink Converter/1 -> Saturation/1
  Saturation/1 -> Z force/1
  connections:
  Floor/RConn1 -- 6-DOF Joint1/LConn1
  6-DOF Joint1/RConn1 -- Contact/RConn1
  No friction/RConn1 -- Y Switch/LConn1 -- Z Switch/LConn1 -- X Switch/LConn1
  Z Position Gain/RConn1 -- Z Add/LConn1
  Z Switch/LConn3 -- PS-Simulink Converter/LConn1 -- Z Add/RConn1 -- Friction coeff/LConn1
  Z Speed Gain/RConn1 -- Z Add/LConn2
  6-DOF Joint1/RConn5 -- Z Speed Gain/LConn1
  6-DOF Joint1/LConn4 -- Z Switch/RConn1
  Z Switch/LConn2 -- Z Position Gain/LConn1 -- 6-DOF Joint1/RConn4 -- X Switch/LConn2 -- Y Switch/LConn2
  Y Switch/RConn1 -- 6-DOF Joint1/LConn3
  Y Speed Gain/LConn1 -- 6-DOF Joint1/RConn3
  PS Abs/LConn1 -- Friction coeff/RConn1
  PS Abs/RConn1 -- Unary minus/LConn1 -- X Upper Bound/LConn2 -- Y Upper Bound/LConn2
  Y Upper Bound/RConn1 -- Y Lower Bound/LConn1
  Y Lower Bound/LConn2 -- Unary minus/RConn1 -- X Lower Bound/LConn2
  Y Lower Bound/RConn1 -- Y Switch/LConn3
  Y Upper Bound/LConn1 -- Y Speed Gain/RConn1
  X Speed Gain/LConn1 -- 6-DOF Joint1/RConn2
  X Upper Bound/LConn1 -- X Speed Gain/RConn1
  X Lower Bound/LConn1 -- X Upper Bound/RConn1
  X Switch/LConn3 -- X Lower Bound/RConn1
  X Switch/RConn1 -- 6-DOF Joint1/LConn2

== system Robot/Robot simulation/Left Leg/Floor model/Floor Model Front Right ==
  6-DOF Joint1 : sm_lib/Joints/6-DOF Joint  SenseConstraintForce=off  SenseConstraintForceX=off  SenseConstraintForceY=off  SenseConstraintForceZ=off  SenseConstraintTorque=off  SenseConstraintTorqueX=off  SenseConstraintTorqueY=off  SenseConstraintTorqueZ=off  SenseTotalForce=off  SenseTotalForceX=off  SenseTotalForceY=off  SenseTotalForceZ=off  SenseTotalTorque=off  SenseTotalTorqueX=off  SenseTotalTorqueY=off  SenseTotalTorqueZ=off  CompositeWrenchDir=FollowerOnBase  CompositeWrenchFrame=BaseFrame  PxEquilibriumPosition=0  PxEquilibriumPositionUnits=m  PxSpringStiffness=0  PxSpringStiffnessUnits=N/m  PxDampingCoefficient=0  PxDampingCoefficientUnits=N/(m/s)  PxTorqueActuationMode=InputTorque  PxMotionActuationMode=ComputedMotion  PxSensePosition=off  PxSenseVelocity=on  PxSenseAcceleration=off  PxSenseTorqueForce=off  PxPositionTargetSpecify=off  PxPositionTargetPriority=High  PxPositionTargetValue=0  PxPositionTargetValueUnits=m  PxVelocityTargetSpecify=off  PxVelocityTargetPriority=High  PxVelocityTargetValue=0  PxVelocityTargetValueUnits=m/s  PyEquilibriumPosition=0  PyEquilibriumPositionUnits=m  PySpringStiffness=0  PySpringStiffnessUnits=N/m  PyDampingCoefficient=0  PyDampingCoefficientUnits=N/(m/s)  PyTorqueActuationMode=InputTorque  PyMotionActuationMode=ComputedMotion  PySensePosition=off  PySenseVelocity=on  PySenseAcceleration=off  PySenseTorqueForce=off  PyPositionTargetSpecify=off  PyPositionTargetPriority=High  PyPositionTargetValue=0  PyPositionTargetValueUnits=m  PyVelocityTargetSpecify=off  PyVelocityTargetPriority=High  PyVelocityTargetValue=0  PyVelocityTargetValueUnits=m/s  PzEquilibriumPosition=0  PzEquilibriumPositionUnits=m  PzSpringStiffness=0  PzSpringStiffnessUnits=N/m  PzDampingCoefficient=0  PzDampingCoefficientUnits=N/(m/s)  PzTorqueActuationMode=InputTorque  PzMotionActuationMode=ComputedMotion  PzSensePosition=on  PzSenseVelocity=on  PzSenseAcceleration=off  PzSenseTorqueForce=off  PzPositionTargetSpecify=off  PzPositionTargetPriority=High  PzPositionTargetValue=0  PzPositionTargetValueUnits=m  PzVelocityTargetSpecify=off  PzVelocityTargetPriority=High  PzVelocityTargetValue=0  PzVelocityTargetValueUnits=m/s  SphDefPosRotationMethod=None  SphDefPosRotationAngleUnits=deg  SphDefPosRotationStandardAxis=+Z  SphDefPosRotationAngle=0.0  SphDefPosRotationArbitraryAxis=[0 0 1]  SphDefPosFollAlignAxisA=+X  SphDefPosBaseAlignAxisA=+Y  SphDefPosFollAlignAxisB=+Y  SphDefPosBaseAlignAxisB=+Z  SphDefPosRotationSequenceAxes=FollowerAxes  SphDefPosRotationSequence=XYX  SphDefPosRotationSequenceAngles=[0 0 0]  SphDefPosRotationSequenceAnglesUnits=deg  SphDefPosRotationMatrix=[1 0 0; 0 1 0; 0 0 1]  SphEqPosRotationMethod=None  SphEqPosRotationAngleUnits=deg  SphEqPosRotationStandardAxis=+Z  SphEqPosRotationAngle=0.0  SphEqPosRotationArbitraryAxis=[0 0 1]  SphEqPosFollAlignAxisA=+X  SphEqPosBaseAlignAxisA=+Y  SphEqPosFollAlignAxisB=+Y  SphEqPosBaseAlignAxisB=+Z  SphEqPosRotationSequenceAxes=FollowerAxes  SphEqPosRotationSequence=XYX  SphEqPosRotationSequenceAngles=[0 0 0]  SphEqPosRotationSequenceAnglesUnits=deg  SphEqPosRotationMatrix=[1 0 0; 0 1 0; 0 0 1]  SphSpringStiffness=0  SphSpringStiffnessUnits=N*m/deg  SphDampingCoefficient=0  SphDampingCoefficientUnits=N*m/(deg/s)  SphActuateTorqueX=off  SphActuateTorqueY=off  SphActuateTorqueZ=off  SphActuateTorque=off  SphTorqueActuationMode=NoTorque  SphMotionActuationMode=ComputedMotion  SphActuationFrame=BaseFrame  SphSensePosition=off  SphSenseVelocityX=off  SphSenseVelocityY=off  SphSenseVelocityZ=off  SphSenseVelocity=off  SphSenseAccelerationX=off  SphSenseAccelerationY=off  SphSenseAccelerationZ=off  SphSenseAcceleration=off  SphSenseTorqueX=off  SphSenseTorqueY=off  SphSenseTorqueZ=off  SphSenseTorqueForce=off  SphSensingFrame=BaseFrame  SphPositionTargetRotationMethod=None  SphPositionTargetRotationAngleUnits=deg  SphPositionTargetRotationStandardAxis=+Z  SphPositionTargetRotationAngle=0.0  SphPositionTargetRotationArbitraryAxis=[0 0 1]  SphPositionTargetFollAlignAxisA=+X  SphPositionTargetBaseAlignAxisA=+Y  SphPositionTargetFollAlignAxisB=+Y  SphPositionTargetBaseAlignAxisB=+Z  SphPositionTargetRotationSequenceAxes=FollowerAxes  SphPositionTargetRotationSequence=XYX  SphPositionTargetRotationSequenceAngles=[0 0 0]  SphPositionTargetRotationSequenceAnglesUnits=deg  SphPositionTargetRotationMatrix=[1 0 0; 0 1 0; 0 0 1]  SphPositionTargetSpecify=off  SphPositionTargetPriority=High  SphVelocityTargetValue=[0 0 0]  SphVelocityTargetValueUnits=deg/s  SphVelocityTargetSpecify=off  SphVelocityTargetPriority=High  SphVelocityTargetInFollowerFrame=on
  Friction coeff : fl_lib/Physical Signals/Functions/PS Gain  gain=robot_floor_friction_coeff
  No friction : fl_lib/Physical Signals/Sources/PS Constant  constant=0
  PS Abs : fl_lib/Physical Signals/Nonlinear Operators/PS Abs
      settings: SourceProductName=Simscape  SourceProductBaseCode=SS
  PS-Simulink Converter : nesl_utility/PS-Simulink Converter  PhysicalDomain=network_engine_domain  SubClassName=ps_output  LeftPortType=input  RightPortType=output  PseudoPeriodic=off  Frequencies=[]  Unit=N  AffineConversion=off
  Saturation : Saturate  UpperLimit=+inf  LowerLimit=0
  Unary minus : fl_lib/Physical Signals/Functions/PS Gain  gain=-1
  X Lower Bound : fl_lib/Physical Signals/Nonlinear Operators/PS Max
      settings: SourceProductName=Simscape  SourceProductBaseCode=SS
  X Speed Gain : fl_lib/Physical Signals/Functions/PS Gain  gain=robot_floor_speed_gain
  X Switch : fl_lib/Physical Signals/Nonlinear Operators/PS Switch  Threshold=0
      settings: SourceProductName=Simscape  SourceProductBaseCode=SS
  X Upper Bound : fl_lib/Physical Signals/Nonlinear Operators/PS Min
      settings: SourceProductName=Simscape  SourceProductBaseCode=SS
  Y Lower Bound : fl_lib/Physical Signals/Nonlinear Operators/PS Max
      settings: SourceProductName=Simscape  SourceProductBaseCode=SS
  Y Speed Gain : fl_lib/Physical Signals/Functions/PS Gain  gain=robot_floor_speed_gain
  Y Switch : fl_lib/Physical Signals/Nonlinear Operators/PS Switch  Threshold=0
      settings: SourceProductName=Simscape  SourceProductBaseCode=SS
  Y Upper Bound : fl_lib/Physical Signals/Nonlinear Operators/PS Min
      settings: SourceProductName=Simscape  SourceProductBaseCode=SS
  Z Add : fl_lib/Physical Signals/Functions/PS Add
  Z Position Gain : fl_lib/Physical Signals/Functions/PS Gain  gain=robot_floor_position_gain
  Z Speed Gain : fl_lib/Physical Signals/Functions/PS Gain  gain=robot_floor_speed_gain
  Z Switch : fl_lib/Physical Signals/Nonlinear Operators/PS Switch  Threshold=0
      settings: SourceProductName=Simscape  SourceProductBaseCode=SS
  Contact : PMIOPort  Side=Left
  Floor : PMIOPort  Port=2  Side=Right
  Z force : Outport
  wires:
  PS-Simulink Converter/1 -> Saturation/1
  Saturation/1 -> Z force/1
  connections:
  Floor/RConn1 -- 6-DOF Joint1/LConn1
  6-DOF Joint1/RConn1 -- Contact/RConn1
  No friction/RConn1 -- Y Switch/LConn1 -- Z Switch/LConn1 -- X Switch/LConn1
  Z Position Gain/RConn1 -- Z Add/LConn1
  Z Switch/LConn3 -- Z Add/RConn1 -- Friction coeff/LConn1 -- PS-Simulink Converter/LConn1
  Z Speed Gain/RConn1 -- Z Add/LConn2
  6-DOF Joint1/RConn5 -- Z Speed Gain/LConn1
  6-DOF Joint1/LConn4 -- Z Switch/RConn1
  Z Switch/LConn2 -- Z Position Gain/LConn1 -- 6-DOF Joint1/RConn4 -- X Switch/LConn2 -- Y Switch/LConn2
  Y Switch/RConn1 -- 6-DOF Joint1/LConn3
  Y Speed Gain/LConn1 -- 6-DOF Joint1/RConn3
  PS Abs/LConn1 -- Friction coeff/RConn1
  PS Abs/RConn1 -- Unary minus/LConn1 -- X Upper Bound/LConn2 -- Y Upper Bound/LConn2
  Y Upper Bound/RConn1 -- Y Lower Bound/LConn1
  Y Lower Bound/LConn2 -- Unary minus/RConn1 -- X Lower Bound/LConn2
  Y Lower Bound/RConn1 -- Y Switch/LConn3
  Y Upper Bound/LConn1 -- Y Speed Gain/RConn1
  X Speed Gain/LConn1 -- 6-DOF Joint1/RConn2
  X Upper Bound/LConn1 -- X Speed Gain/RConn1
  X Lower Bound/LConn1 -- X Upper Bound/RConn1
  X Switch/LConn3 -- X Lower Bound/RConn1
  X Switch/RConn1 -- 6-DOF Joint1/LConn2
